simulink model "plant_model_bicycle"  (R2021b)
settings: Solver=VariableStepAuto  StartTime=0.0  StopTime=10.0  RelTol=1e-3
values from neighbouring files (symbols this model uses):
  desired_lateral_position = 0.1    [simulation_results.m]
  PID_derivative_gain = 10    [simulation_results.m]
  PID_integration_gain = 0.02    [simulation_results.m]
  PID_proportional_gain = 3    [simulation_results.m]
  steering_wheel_angle = 3    [simulation_results.m]
settings Model: Creator=kacsk  LastModifiedBy=kacsk

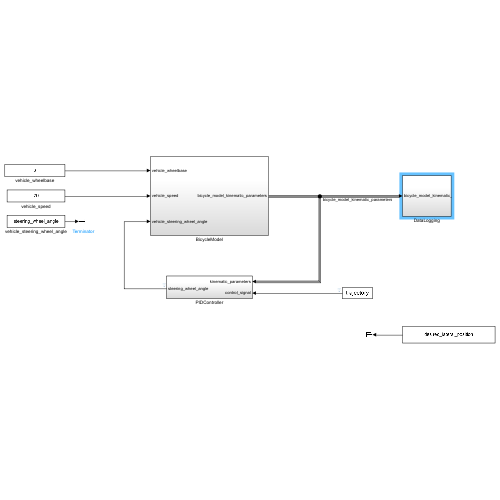
[thumbnail: Simulink's stored preview of the top-level diagram]
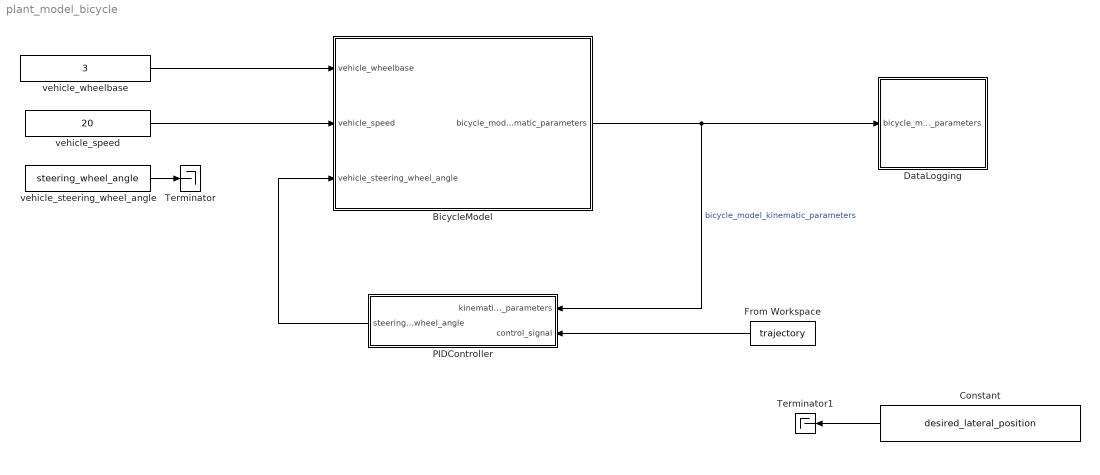
== system plant_model_bicycle ==
  BicycleModel : Subsystem
  Constant : Constant  Value=desired_lateral_position
  DataLogging : Subsystem
  From Workspace : FromWorkspace  VariableName=trajectory  SampleTime=0.1
  PIDController : Subsystem
  Terminator : Terminator
  Terminator1 : Terminator
  vehicle_speed : Constant  Value=20
  vehicle_steering_wheel_angle : Constant  Value=steering_wheel_angle
  vehicle_wheelbase : Constant  Value=3
  wires:
  vehicle_wheelbase/1 -> BicycleModel/1(vehicle_wheelbase)
  vehicle_speed/1 -> BicycleModel/2(vehicle_speed)
  BicycleModel/1(bicycle_model_kinematic_parameters) -> PIDController/1(kinematic_parameters), DataLogging/1(bicycle_model_kinematic_parameters)  "bicycle_model_kinematic_parameters"
  From Workspace/1 -> PIDController/2(control_signal)
  vehicle_steering_wheel_angle/1 -> Terminator/1
  PIDController/1(steering_wheel_angle) -> BicycleModel/3(vehicle_steering_wheel_angle)
  Constant/1 -> Terminator1/1

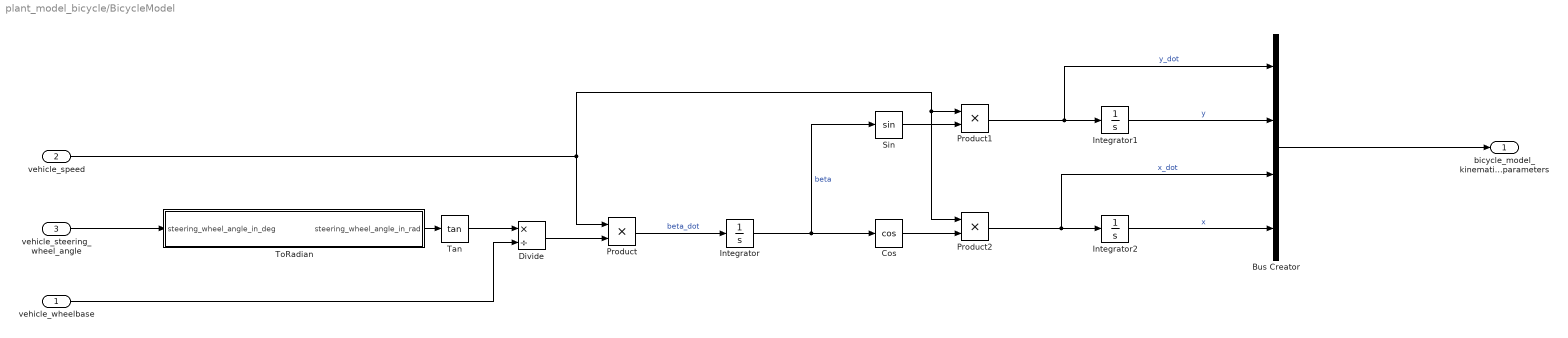
== system plant_model_bicycle/BicycleModel ==
  vehicle_wheelbase : Inport
  vehicle_speed : Inport  Port=2
  vehicle_steering_wheel_angle : Inport  Port=3
  Bus Creator : BusCreator  Inputs=4
  Cos : Trigonometry  Operator=cos
  Divide : Product  Inputs=*/
  Integrator : Integrator
  Integrator1 : Integrator
  Integrator2 : Integrator
  Product : Product
  Product1 : Product
  Product2 : Product
  Sin : Trigonometry
  Tan : Trigonometry  Operator=tan
  ToRadian : Subsystem
  bicycle_model_kinematic_parameters : Outport
  wires:
  Tan/1 -> Divide/1
  vehicle_wheelbase/1 -> Divide/2
  Divide/1 -> Product/2
  vehicle_speed/1 -> Product2/1, Product1/1, Product/1
  Product/1 -> Integrator/1  "beta_dot"
  Integrator/1 -> Sin/1, Cos/1  "beta"
  Sin/1 -> Product1/2
  Product1/1 -> Bus Creator/1, Integrator1/1  "y_dot"
  Cos/1 -> Product2/2
  Product2/1 -> Bus Creator/3, Integrator2/1  "x_dot"
  Integrator2/1 -> Bus Creator/4  "x"
  Integrator1/1 -> Bus Creator/2  "y"
  Bus Creator/1 -> bicycle_model_kinematic_parameters/1
  ToRadian/1(steering_wheel_angle_in_rad) -> Tan/1
  vehicle_steering_wheel_angle/1 -> ToRadian/1(steering_wheel_angle_in_deg)

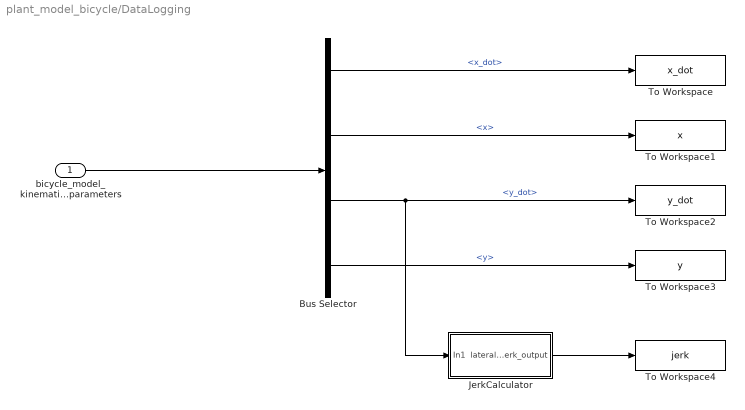
== system plant_model_bicycle/DataLogging ==
  bicycle_model_kinematic_parameters : Inport
  Bus Selector : BusSelector  OutputSignals=x_dot,x,y_dot,y
  JerkCalculator : Subsystem
  To Workspace : ToWorkspace  VariableName=x_dot  SampleTime=-1
  To Workspace1 : ToWorkspace  VariableName=x  SampleTime=-1
  To Workspace2 : ToWorkspace  VariableName=y_dot  SampleTime=-1
  To Workspace3 : ToWorkspace  VariableName=y  SampleTime=-1
  To Workspace4 : ToWorkspace  VariableName=jerk  SampleTime=-1
  wires:
  bicycle_model_kinematic_parameters/1 -> Bus Selector/1
  Bus Selector/1 -> To Workspace/1  "<x_dot>"
  Bus Selector/2 -> To Workspace1/1  "<x>"
  Bus Selector/3 -> JerkCalculator/1(In1), To Workspace2/1  "<y_dot>"
  Bus Selector/4 -> To Workspace3/1  "<y>"
  JerkCalculator/1(lateral_jerk_output) -> To Workspace4/1

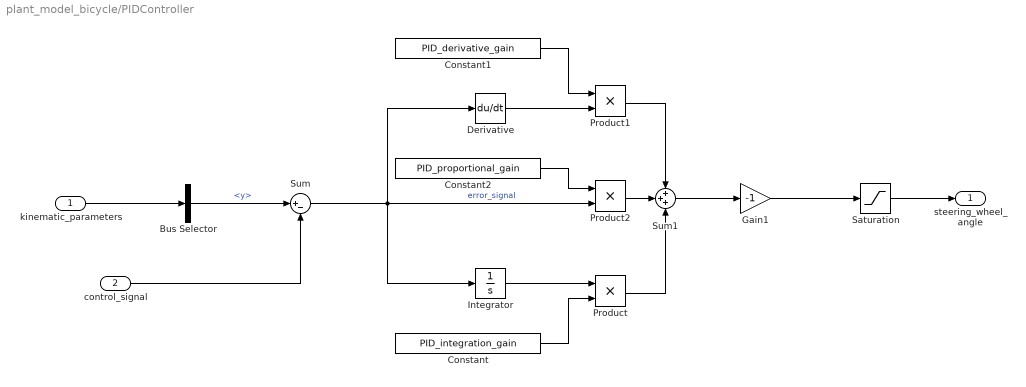
== system plant_model_bicycle/PIDController ==
  kinematic_parameters : Inport
  control_signal : Inport  Port=2
  Bus Selector : BusSelector  OutputSignals=y
  Constant : Constant  Value=PID_integration_gain
  Constant1 : Constant  Value=PID_derivative_gain
  Constant2 : Constant  Value=PID_proportional_gain
  Derivative : Derivative
  Gain1 : Gain  Gain=-1
  Integrator : Integrator
  Product : Product
  Product1 : Product
  Product2 : Product
  Saturation : Saturate  UpperLimit=10  LowerLimit=-10
  Sum : Sum  Inputs=|+-
  Sum1 : Sum  Inputs=+++
  steering_wheel_angle : Outport
  wires:
  control_signal/1 -> Sum/2
  kinematic_parameters/1 -> Bus Selector/1
  Bus Selector/1 -> Sum/1  "<y>"
  Sum/1 -> Product2/2, Integrator/1, Derivative/1  "error_signal"
  Product2/1 -> Sum1/2
  Gain1/1 -> Saturation/1
  Integrator/1 -> Product/1
  Sum1/1 -> Gain1/1
  Product/1 -> Sum1/3
  Derivative/1 -> Product1/2
  Product1/1 -> Sum1/1
  Saturation/1 -> steering_wheel_angle/1
  Constant/1 -> Product/2
  Constant1/1 -> Product1/1
  Constant2/1 -> Product2/1

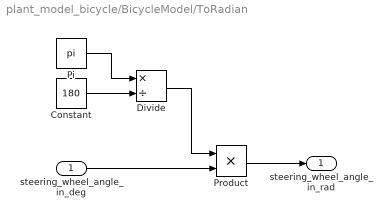
== system plant_model_bicycle/BicycleModel/ToRadian ==
  steering_wheel_angle_in_deg : Inport
  Constant : Constant  Value=180
  Divide : Product  Inputs=*/
  Pi : Constant  Value=pi  OutDataTypeStr=Inherit: Inherit via back propagation
  Product : Product
  steering_wheel_angle_in_rad : Outport
  wires:
  Pi/1 -> Divide/1
  Constant/1 -> Divide/2
  Divide/1 -> Product/1
  steering_wheel_angle_in_deg/1 -> Product/2
  Product/1 -> steering_wheel_angle_in_rad/1

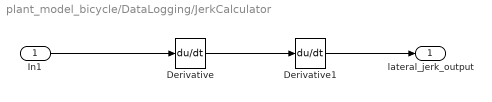
== system plant_model_bicycle/DataLogging/JerkCalculator ==
  In1 : Inport
  Derivative : Derivative
  Derivative1 : Derivative
  lateral_jerk_output : Outport
  wires:
  Derivative/1 -> Derivative1/1
  In1/1 -> Derivative/1
  Derivative1/1 -> lateral_jerk_output/1
